simulink model "lecture8_simplemat"  (Simulink 7.1)
settings: Solver=FixedStepDiscrete  StartTime=0.0  StopTime=10.0  RelTol=1e-3
settings Model: Creator=pit  LastModifiedBy=pit

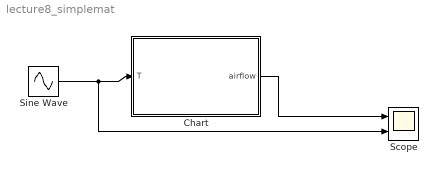
== system lecture8_simplemat ==
  Chart : Stateflow chart
  Scope : Scope  NumInputPorts=2
      settings: YMin=-5~-5  YMax=5~5
  Sine Wave : Sin  Amplitude=50  SampleTime=0
  wires:
  Sine Wave/1 -> Chart/1(T), Scope/2
  Chart/1(airflow) -> Scope/1

== stateflow chart Chart ==
  state Off
    during: airflow=0
  state On
    during:airflow=1
  Off -> On : [T < 10]
  On -> Off : [T > 20+ml.rand()]
  (default) -> Off
  data: airflow output double; T input double
